simulink model "CartPoleMathworksModified"  (R2022b)
settings: Solver=ode45  StartTime=0  StopTime=ESSettings.tend  MaxStep=0.02  RelTol=1e-3  AbsTol=1e-6
undefined symbols (not defined in the file or in its folder): CtrlSettings
libraries: UtilLib x1
Description:
  | Inverted Pendulum with Animation
  | 
  | This example shows how to model an inverted pendulum.  The animation is created using MATLAB(R) Handle Graphics(R).  The animation block is a masked
  | S-function.  For more information, use the context menu to look under the Animation block's mask
  | and open the S-function for editing.
settings Model: Creator=The MathWorks, Inc.  LastModifiedBy=vd818225
settings SolverCC: AutoScaleAbsTol=off  AlgebraicLoopSolver=TrustRegion
settings DataIOCC: ExternalInput=[]  InitialState=[]  SaveFormat=Array  SaveOutput=off  SaveTime=off
settings OptimizationCC: BlockReduction=off  BooleanDataType=off  ExpressionDepthLimit=2147483647  InitFltsAndDblsToZero=on  LifeSpan=inf
settings DebuggingCC: SaveWithParameterizedLinksMsg=none  UnderspecifiedInitializationDetection=Classic  MergeDetectMultiDrivingBlocksExec=none  SignalResolutionControl=TryResolveAllWithWarning  MultiTaskDSMMsg=warning  MultiTaskCondExecSysMsg=none  SigSpecEnsureSampleTimeMsg=none  FcnCallInpInsideContextMsg=warning  UnconnectedInputMsg=warning  UnconnectedOutputMsg=warning  UnconnectedLineMsg=warning  StateNameClashWarn=warning  SFUnexpectedBacktrackingDiag=warning  SFNoUnconditionalDefaultTransitionDiag=warning  SFExecutionAtInitializationDiag=none  SFMachineParentedDataDiag=warning  ArithmeticOperatorsInVariantConditions=warning
settings HardwareCC: ProdBitPerPointer=32  ProdBitPerSizeT=32  ProdBitPerPtrDiffT=32  ProdLargestAtomicFloat=None  ProdIntDivRoundTo=Undefined  ProdEndianess=Unspecified  ProdWordSize=32  ProdHWDeviceType=32-bit Generic  TargetUnknown=on
settings ModelReferenceCC: EnableRefExpFcnMdlSchedulingChecks=on  PropagateSignalLabelsOutOfModel=off
settings SFSimCC: SimUseLocalCustomCode=off  CustomCodeUndefinedFunction=UseInterfaceOnly
settings RTWCC: RTWUseLocalCustomCode=off
settings CodeAppCC: StateflowObjectComments=on
settings GRTTargetCC: TargetFcnLib=ansi_tfl_tmw.mat  TargetLangStandard=C89/C90 (ANSI)  CombineOutputUpdateFcns=off  GRTInterface=on
settings ConfigComp: CovMetricSettings=dw  CovSaveCumulativeToWorkspaceVar=on  CovSaveSingleToWorkspaceVar=on  CovExternalEMLEnable=off

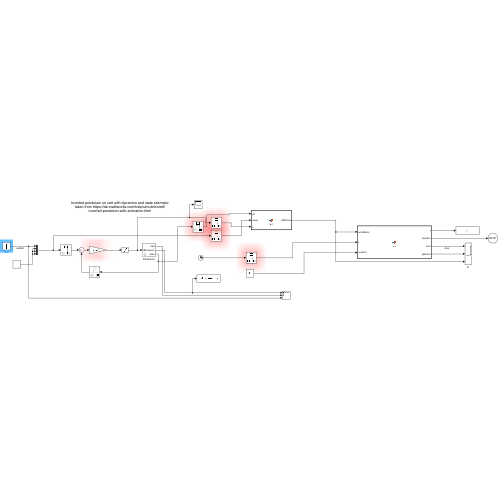
[thumbnail: Simulink's stored preview of the top-level diagram]
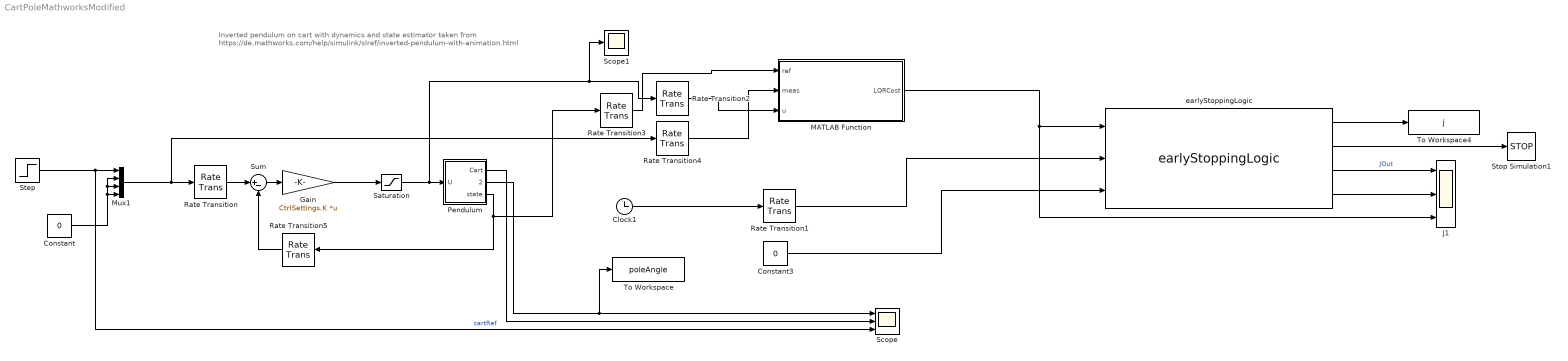
== system CartPoleMathworksModified ==
  note: Inverted pendulum on cart with dynamics and state estimator taken from https://de.mathworks.com/help/simulink/slref/inverted-pendulum-with-animation.html
  Clock1 : Clock
  Constant : Constant  Value=0
  Constant3 : Constant  Value=0
  Gain : Gain  Gain=CtrlSettings.K  Multiplication=Matrix(K*u) (u vector)
  J1 : Scope  NumInputPorts=3
  MATLAB Function : MATLAB Function  TreatAsAtomicUnit=on
  Mux1 : Mux
  Pendulum : Subsystem  mask(Inverted pendulum on cart){Mcart=0.455, m=0.21, l=0.61/2, g=9.8}
      mask prompts: Mcart "Mass of cart (kg):"; m "Mass of pendulum (kg):"; l "Distance to pendulum center of mass(m):"; g "Acceleration of gravity (m/s^2):"
      mask help: Unmask and double-click to see dynamics
      mask Help: Nonlinear dynamics of inverted pendulum on cart.
  Rate Transition : RateTransition  OutPortSampleTime=0.02
  Rate Transition{1..4} (4 alike) : RateTransition  OutPortSampleTime=ESSettings.t_obj
  Rate Transition5 : RateTransition  OutPortSampleTime=0.02
  Saturation : Saturate  UpperLimit=10  LowerLimit=-10
  Scope : Scope  NumInputPorts=3
  Scope1 : Scope
  Step : Step  Time=10  SampleTime=0
  Stop Simulation1 : Stop
  Sum : Sum  Inputs=|+-
  To Workspace : ToWorkspace  VariableName=poleAngle  SaveFormat=Timeseries  SampleTime=-1
  To Workspace4 : ToWorkspace  VariableName=j  SaveFormat=Structure With Time  SampleTime=-1
  earlyStoppingLogic : UtilLib/earlyStoppingLogic  SystemSampleTime=-1  VariantActivationTime=update diagram  Latency=0  AutoFrameSizeCalculation=off
  wires:
  Pendulum/3(state) -> Rate Transition5/1, Rate Transition3/1
  Pendulum/2(Pendulum) -> To Workspace/1, Scope/1
  Pendulum/1(Cart) -> Scope/2
  Step/1 -> Scope/3, Mux1/1  "cartRef"
  Sum/1 -> Gain/1
  Mux1/1 -> Rate Transition4/1, Rate Transition/1
  Constant/1 -> Mux1/2, Mux1/3, Mux1/4
  earlyStoppingLogic/4 -> J1/2
  earlyStoppingLogic/1 -> To Workspace4/1
  earlyStoppingLogic/3 -> J1/1  "JOut"
  MATLAB Function/1(LQRCost) -> J1/3, earlyStoppingLogic/1
  Clock1/1 -> Rate Transition1/1
  earlyStoppingLogic/2 -> Stop Simulation1/1
  Constant3/1 -> earlyStoppingLogic/3
  Rate Transition3/1 -> MATLAB Function/1(ref)
  Rate Transition4/1 -> MATLAB Function/2(meas)
  Rate Transition1/1 -> earlyStoppingLogic/2
  Saturation/1 -> Scope1/1, Rate Transition2/1, Pendulum/1(U)
  Rate Transition/1 -> Sum/1
  Rate Transition2/1 -> MATLAB Function/3(u)
  Gain/1 -> Saturation/1
  Rate Transition5/1 -> Sum/2

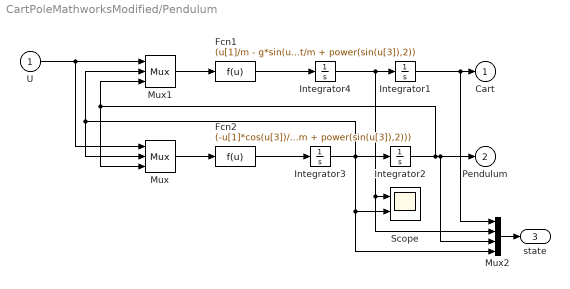
== system CartPoleMathworksModified/Pendulum ==
  U : Inport
  Fcn1 : Fcn  Expr=(u[1]/m - g*sin(u[3])*cos(u[3]) + l*power(u[2],2)*sin(u[3]))/(Mcart/m + power(sin(u[3]),2))
  Fcn2 : Fcn  Expr=(-u[1]*cos(u[3])/m + (Mcart+m)*g*sin(u[3])/m - l*power(u[2],2)*sin(u[3])*cos(u[3]))/(l*(Mcart/m + power(sin(u[3]),2)))
  Integrator1 : Integrator  UpperSaturationLimit=3  LowerSaturationLimit=-3
  Integrator2 : Integrator  InitialCondition=30/180*pi
  Integrator3 : Integrator
  Integrator4 : Integrator
  Mux : Mux  Inputs=3
  Mux1 : Mux  Inputs=3
  Mux2 : Mux
  Scope : Scope  NumInputPorts=2
  Cart : Outport  InitialOutput=0  VectorParamsAs1DForOutWhenUnconnected=off
  Pendulum : Outport  Port=2  InitialOutput=0  VectorParamsAs1DForOutWhenUnconnected=off
  state : Outport  Port=3
  wires:
  Integrator1/1 -> Mux2/1, Cart/1
  Fcn2/1 -> Integrator3/1
  Mux/1 -> Fcn2/1
  Mux1/1 -> Fcn1/1
  Fcn1/1 -> Integrator4/1
  Integrator4/1 -> Mux2/2, Scope/1, Integrator1/1
  U/1 -> Mux1/1, Mux/1
  Integrator3/1 -> Scope/2, Mux2/4, Integrator2/1, Mux1/2, Mux/2
  Integrator2/1 -> Pendulum/1, Mux2/3, Mux1/3, Mux/3
  Mux2/1 -> state/1

== matlab function CartPoleMathworksModified/MATLAB Function ==
  data: ref input; LQRCost output; meas input; u input; CostMat parameter
function LQRCost  = fcn(ref, meas,u,CostMat)
LQRCost = sum(abs(min(abs(ref-meas),2)).^2.*CostMat.R' + u.^2*CostMat.Q);
end
